simulink model "koen_q_axis_current_loop_model"  (R2024b)
settings: Solver=FixedStepDiscrete  StartTime=0.0  StopTime=0.02  FixedStep=6.25e-05  RelTol=1e-3
PreLoadFcn:
  | FOC_TS_SEC=6.25e-05; FOC_IQ_KP=3.77; FOC_IQ_KI=3330; FOC_CURR_LOOP_V_LIMIT=13.5; FOC_DQ_VOLT_LIMIT=13.5; FOC_VQ_CMD_SIGN=-1; FOC_RS_OHM=0.53; FOC_LQ_H=0.0006; FOC_FLUX_WB=0.0078; OMEGA_E_RAD_S=0;
undefined symbols (not defined in the file or in its folder): DiscIntNeverNeededParam
settings Model: Creator=10095  LastModifiedBy=10095

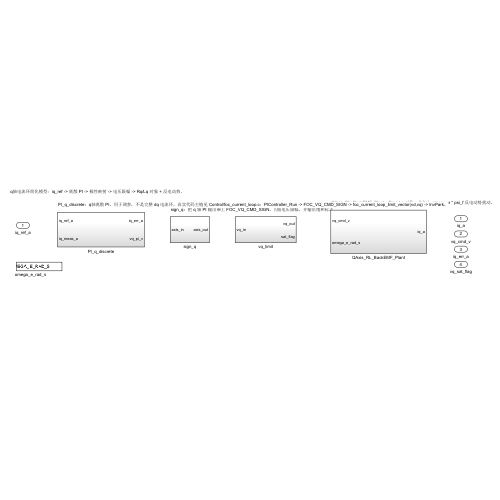
[thumbnail: Simulink's stored preview of the top-level diagram]
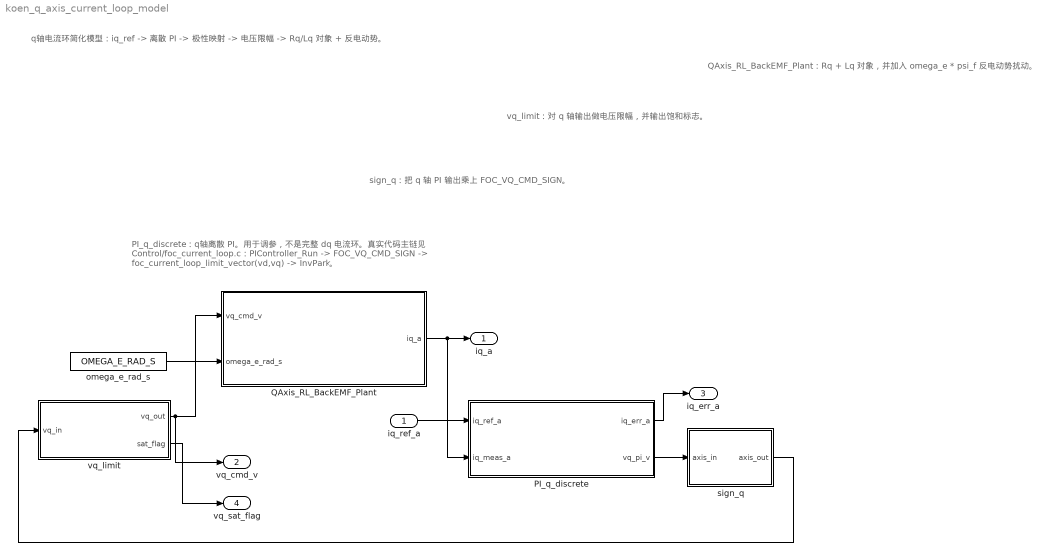
== system koen_q_axis_current_loop_model ==
  note: PI_q_discrete：q轴离散 PI。用于调参，不是完整 dq 电流环。真实代码主链见 Control/foc_current_loop.c：PIController_Run -> FOC_VQ_CMD_SIGN -> foc_current_loop_limit_vector(vd,vq) -> InvPark。
  note: sign_q：把 q 轴 PI 输出乘上 FOC_VQ_CMD_SIGN。
  note: vq_limit：对 q 轴输出做电压限幅，并输出饱和标志。
  note: QAxis_RL_BackEMF_Plant：Rq + Lq 对象，并加入 omega_e * psi_f 反电动势扰动。
  note: q轴电流环简化模型：iq_ref -> 离散 PI -> 极性映射 -> 电压限幅 -> Rq/Lq 对象 + 反电动势。
  iq_ref_a : Inport
  PI_q_discrete : Subsystem  Description=PI_q_discrete：q轴离散 PI。用于调参，不是完整 dq 电流环。真实代码主链见 Control/foc_current_loop.c：PIController_Run -> FOC_VQ_CMD_SIGN -> foc_current_loop_limit_vector(vd,vq) -> InvPark。
  QAxis_RL_BackEMF_Plant : Subsystem  Description=QAxis_RL_BackEMF_Plant：Rq + Lq 对象，并加入 omega_e * psi_f 反电动势扰动。
  omega_e_rad_s : Constant  Value=OMEGA_E_RAD_S
  sign_q : Subsystem  Description=sign_q：把 q 轴 PI 输出乘上 FOC_VQ_CMD_SIGN。
  vq_limit : Subsystem  Description=vq_limit：对 q 轴输出做电压限幅，并输出饱和标志。
  iq_a : Outport
  vq_cmd_v : Outport  Port=2
  iq_err_a : Outport  Port=3
  vq_sat_flag : Outport  Port=4
  wires:
  vq_limit/2(sat_flag) -> vq_sat_flag/1
  vq_limit/1(vq_out) -> vq_cmd_v/1, QAxis_RL_BackEMF_Plant/1(vq_cmd_v)
  omega_e_rad_s/1 -> QAxis_RL_BackEMF_Plant/2(omega_e_rad_s)
  QAxis_RL_BackEMF_Plant/1(iq_a) -> PI_q_discrete/2(iq_meas_a), iq_a/1
  PI_q_discrete/2(vq_pi_v) -> sign_q/1(axis_in)
  PI_q_discrete/1(iq_err_a) -> iq_err_a/1
  iq_ref_a/1 -> PI_q_discrete/1(iq_ref_a)
  sign_q/1(axis_out) -> vq_limit/1(vq_in)

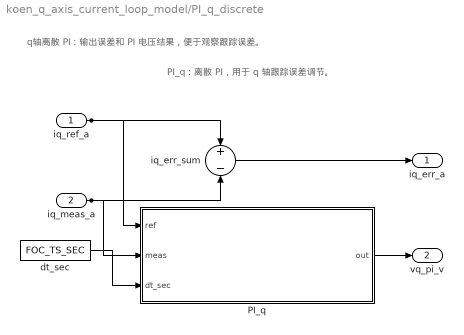
== system koen_q_axis_current_loop_model/PI_q_discrete ==
  note: PI_q：离散 PI，用于 q 轴跟踪误差调节。
  note: q轴离散 PI：输出误差和 PI 电压结果，便于观察跟踪误差。
  iq_ref_a : Inport
  iq_meas_a : Inport  Port=2
  PI_q : Subsystem  Description=PI_q：离散 PI，用于 q 轴跟踪误差调节。
  dt_sec : Constant  Value=FOC_TS_SEC
  iq_err_sum : Sum  Inputs=+-
  iq_err_a : Outport
  vq_pi_v : Outport  Port=2
  wires:
  iq_meas_a/1 -> iq_err_sum/2, PI_q/2(meas)
  iq_ref_a/1 -> iq_err_sum/1, PI_q/1(ref)
  dt_sec/1 -> PI_q/3(dt_sec)
  PI_q/1(out) -> vq_pi_v/1
  iq_err_sum/1 -> iq_err_a/1

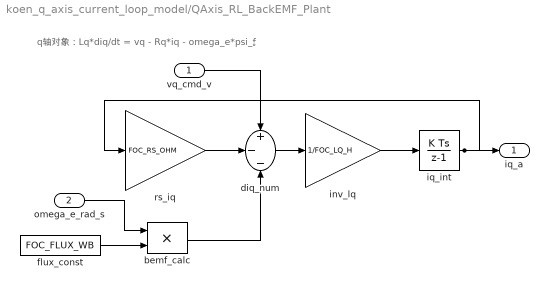
== system koen_q_axis_current_loop_model/QAxis_RL_BackEMF_Plant ==
  note: q轴对象：Lq*diq/dt = vq - Rq*iq - omega_e*psi_f。
  vq_cmd_v : Inport
  omega_e_rad_s : Inport  Port=2
  bemf_calc : Product
  diq_num : Sum  Inputs=+--
  flux_const : Constant  Value=FOC_FLUX_WB
  inv_lq : Gain  Gain=1/FOC_LQ_H
  iq_int : DiscreteIntegrator  SampleTime=FOC_TS_SEC  ICPrevOutput=DiscIntNeverNeededParam  ICPrevScaledInput=DiscIntNeverNeededParam
  rs_iq : Gain  Gain=FOC_RS_OHM
  iq_a : Outport
  wires:
  vq_cmd_v/1 -> diq_num/1
  omega_e_rad_s/1 -> bemf_calc/1
  iq_int/1 -> rs_iq/1, iq_a/1
  inv_lq/1 -> iq_int/1
  diq_num/1 -> inv_lq/1
  bemf_calc/1 -> diq_num/3
  rs_iq/1 -> diq_num/2
  flux_const/1 -> bemf_calc/2

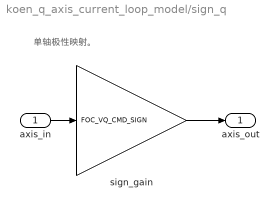
== system koen_q_axis_current_loop_model/sign_q ==
  note: 单轴极性映射。
  axis_in : Inport
  sign_gain : Gain  Gain=FOC_VQ_CMD_SIGN
  axis_out : Outport
  wires:
  sign_gain/1 -> axis_out/1
  axis_in/1 -> sign_gain/1

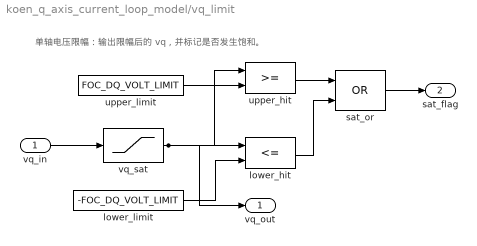
== system koen_q_axis_current_loop_model/vq_limit ==
  note: 单轴电压限幅：输出限幅后的 vq，并标记是否发生饱和。
  vq_in : Inport
  lower_hit : RelationalOperator  Operator=<=  OutDataTypeStr=boolean  RndMeth=Simplest  InputSameDT=off
  lower_limit : Constant  Value=-FOC_DQ_VOLT_LIMIT
  sat_or : Logic  Operator=OR  AllPortsSameDT=off  OutDataTypeStr=boolean
  upper_hit : RelationalOperator  OutDataTypeStr=boolean  RndMeth=Simplest  InputSameDT=off
  upper_limit : Constant  Value=FOC_DQ_VOLT_LIMIT
  vq_sat : Saturate  UpperLimit=FOC_DQ_VOLT_LIMIT  LowerLimit=-FOC_DQ_VOLT_LIMIT
  vq_out : Outport
  sat_flag : Outport  Port=2
  wires:
  vq_sat/1 -> upper_hit/1, vq_out/1, lower_hit/1
  vq_in/1 -> vq_sat/1
  sat_or/1 -> sat_flag/1
  lower_limit/1 -> lower_hit/2
  upper_limit/1 -> upper_hit/2
  lower_hit/1 -> sat_or/2
  upper_hit/1 -> sat_or/1

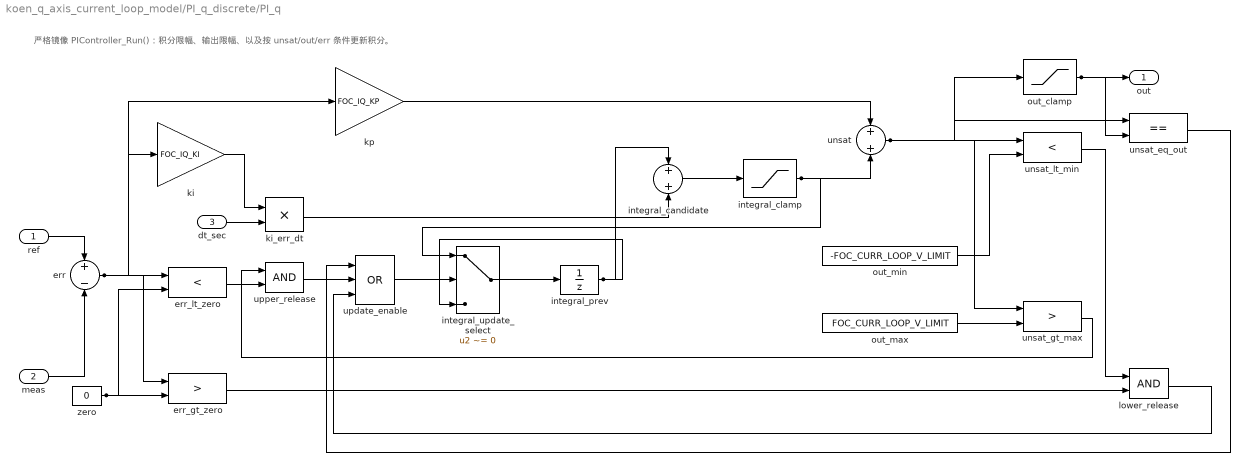
== system koen_q_axis_current_loop_model/PI_q_discrete/PI_q ==
  note: 严格镜像 PIController_Run()：积分限幅、输出限幅、以及按 unsat/out/err 条件更新积分。
  ref : Inport
  meas : Inport  Port=2
  dt_sec : Inport  Port=3
  err : Sum  Inputs=+-
  err_gt_zero : RelationalOperator  Operator=>  OutDataTypeStr=boolean  RndMeth=Simplest  InputSameDT=off
  err_lt_zero : RelationalOperator  Operator=<  OutDataTypeStr=boolean  RndMeth=Simplest  InputSameDT=off
  integral_candidate : Sum
  integral_clamp : Saturate  UpperLimit=FOC_CURR_LOOP_V_LIMIT  LowerLimit=-FOC_CURR_LOOP_V_LIMIT
  integral_prev : UnitDelay  SampleTime=FOC_TS_SEC  HasFrameUpgradeWarning=on
  integral_update_select : Switch  Criteria=u2 ~= 0  Threshold=0.5  SaturateOnIntegerOverflow=off  InputSameDT=off
  ki : Gain  Gain=FOC_IQ_KI
  ki_err_dt : Product
  kp : Gain  Gain=FOC_IQ_KP
  lower_release : Logic  AllPortsSameDT=off  OutDataTypeStr=boolean
  out_clamp : Saturate  UpperLimit=FOC_CURR_LOOP_V_LIMIT  LowerLimit=-FOC_CURR_LOOP_V_LIMIT
  out_max : Constant  Value=FOC_CURR_LOOP_V_LIMIT
  out_min : Constant  Value=-FOC_CURR_LOOP_V_LIMIT
  unsat : Sum
  unsat_eq_out : RelationalOperator  Operator===  OutDataTypeStr=boolean  RndMeth=Simplest  InputSameDT=off
  unsat_gt_max : RelationalOperator  Operator=>  OutDataTypeStr=boolean  RndMeth=Simplest  InputSameDT=off
  unsat_lt_min : RelationalOperator  Operator=<  OutDataTypeStr=boolean  RndMeth=Simplest  InputSameDT=off
  update_enable : Logic  Operator=OR  Inputs=3  AllPortsSameDT=off  OutDataTypeStr=boolean
  upper_release : Logic  AllPortsSameDT=off  OutDataTypeStr=boolean
  zero : Constant  Value=0
  out : Outport
  wires:
  meas/1 -> err/2
  ref/1 -> err/1
  ki/1 -> ki_err_dt/1
  err/1 -> kp/1, ki/1, err_lt_zero/1, err_gt_zero/1
  out_max/1 -> unsat_gt_max/2
  zero/1 -> err_lt_zero/2, err_gt_zero/2
  dt_sec/1 -> ki_err_dt/2
  upper_release/1 -> update_enable/2
  err_lt_zero/1 -> upper_release/2
  err_gt_zero/1 -> lower_release/2
  integral_candidate/1 -> integral_clamp/1
  ki_err_dt/1 -> integral_candidate/2
  kp/1 -> unsat/1
  update_enable/1 -> integral_update_select/2
  integral_update_select/1 -> integral_prev/1
  integral_prev/1 -> integral_update_select/3, integral_candidate/1
  unsat/1 -> unsat_eq_out/1, out_clamp/1, unsat_gt_max/1, unsat_lt_min/1
  integral_clamp/1 -> integral_update_select/1, unsat/2
  unsat_gt_max/1 -> upper_release/1
  unsat_lt_min/1 -> lower_release/1
  out_min/1 -> unsat_lt_min/2
  out_clamp/1 -> out/1, unsat_eq_out/2
  unsat_eq_out/1 -> update_enable/1
  lower_release/1 -> update_enable/3
